simulink model "microgrid_phasor"  (R2025a)
settings: Solver=ode23tb  StartTime=0  StopTime=4253.748  RelTol=1e-4
libraries: spsGroundLib x3, spsThreePhaseParallelRLCBranchLib x1, spsThreePhaseDynamicLoadLib x1, spsThreePhaseSourceLib x1, spsThreePhaseVIMeasurementLib x1, spspowerguiLib x1
settings Model: Creator=daniellee  LastModifiedBy=daniellee

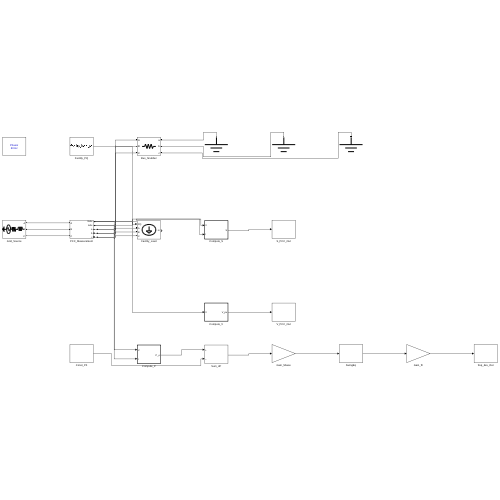
[thumbnail: Simulink's stored preview of the top-level diagram]
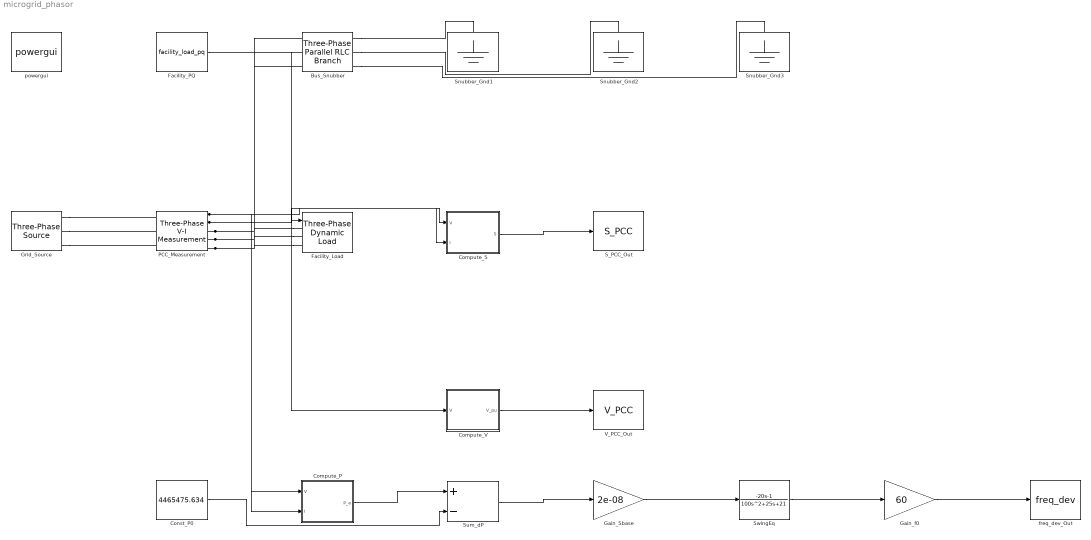
== system microgrid_phasor ==
  Bus_Snubber : spsThreePhaseParallelRLCBranchLib/Three-Phase Parallel RLC Branch  LConnTagsString=A|B|C  RConnTagsString=A|B|C  BranchType=R  Resistance=1e7  Inductance=1e9  Capacitance=1e-12  Measurements=None
  Compute_P : MATLAB Function  TreatAsAtomicUnit=on
  Compute_S : MATLAB Function  TreatAsAtomicUnit=on
  Compute_V : MATLAB Function  TreatAsAtomicUnit=on
  Const_P0 : Constant  Value=4465475.634
  Facility_Load : spsThreePhaseDynamicLoadLib/Three-Phase Dynamic Load  NominalVoltage=[25000 60]  ActiveReactivePowers=[4465475.634 1275123.081]  PositiveSequence=[0.994 -11.8]  ExternalControl=on  NpNq=[0 0]  TimeConstants="[0  0  0  0]"  MinimumVoltage=0.7  Tfilter=1e-4  LoadFlowParameters=[4,0,0,0,0]
      settings: LibrarySourceBlock=|
      | sps_lib/Passives/Three-Phase
      | Dynamic Load
  Facility_PQ : FromWorkspace  VariableName=facility_load_pq  OutputAfterFinalValue=Holding final value
  Gain_Sbase : Gain  Gain=2e-08
  Gain_f0 : Gain  Gain=60
  Grid_Source : spsThreePhaseSourceLib/Three-Phase Source  InternalConnection=Yg  VoltagePhases=off  Voltage=25000  PhaseAngle=0  Voltage_phases=[25e3 25e3 25e3]/sqrt(3)  PhaseAngles_phases=[0 -120 +120]  Frequency=60  NonIdealSource=on  SpecifyImpedance=on  Resistance=0.8929  Inductance=16.58e-3  ShortCircuitLevel=100000000  BaseVoltage=25000  XRratio=7  BusType=swing  Pref=10e3  Qref=0  Prefabc=[10e3, 10e3, 10e3]  Qrefabc=[0, 0, 0]  Qmin=-inf  Qmax=inf
  PCC_Measurement : spsThreePhaseVIMeasurementLib/Three-Phase V-I Measurement  VoltageMeasurement=phase-to-ground  SetLabelV=off  LabelV=Vabc  Vpu=off  VpuLL=off  CurrentMeasurement=yes  SetLabelI=off  LabelI=Iabc  Ipu=off  Pbase=100e6  Vbase=500e3  OutputType=Complex  PhasorSimulation=off  PSBequivalent=0
  S_PCC_Out : ToWorkspace  VariableName=S_PCC  SaveFormat=Timeseries  SampleTime=-1
  Snubber_Gnd1 : spsGroundLib/Ground  LConnTagsString=a
  Snubber_Gnd2 : spsGroundLib/Ground  LConnTagsString=a
  Snubber_Gnd3 : spsGroundLib/Ground  LConnTagsString=a
  Sum_dP : Sum  Inputs=+-
  SwingEq : TransferFcn  Numerator=[-20 -1]  Denominator=[100 25 21]
  V_PCC_Out : ToWorkspace  VariableName=V_PCC  SaveFormat=Timeseries  SampleTime=-1
  freq_dev_Out : ToWorkspace  VariableName=freq_dev  SaveFormat=Timeseries  SampleTime=-1
  powergui : spspowerguiLib/powergui  Priority=1  SimulationMode=Phasor  SampleTime=50e-6  frequency=60  Iterations=50  frequencyindice=60  Pbase=100e6  ErrMax=1e-4  UnitsV=kV  UnitsW=MW  buscounter=0  FunctionMessages=off  echomessages=off  EnableUseOfTLC=off  CurrentSourceSwitches=off  DisableSnubberDevices=off  DisableRonSwitches=off  DisableVfSwitches=off  DisplayEquations=off  AutomaticDiscreteSolvers=off  SolverType=Tustin/Backward Euler (TBE)  Interpol=off  ExternalGateDelay=off  methode=off  Ts=100  x0status=blocks  SPID=on  SwTol=0  HookPort=off  NonlinearTolerance=1e-4  nMaxIteration=100  ContinueOnMaxIteration=off  RestoreLinks=warning  ResistiveCurrentMeasurement=off  Frange=[0:2:500]  Ylog=off  Xlog=on  ShowGrid=off  save=off  variable=ZData  structure=0  ZoomFFT=off  StartTime=0.0  cycles=1  DisplayStyle=1  fundamental=60  FreqAxis=off  MaxFrequency=1000  frequencyindicesteady=1  RmsSteady=1  display=off
  wires:
  Facility_PQ/1 -> Facility_Load/1
  PCC_Measurement/1 -> Compute_S/1(V), Compute_V/1(V), Compute_P/1(V)
  PCC_Measurement/2 -> Compute_S/2(I), Compute_P/2(I)
  Compute_S/1(S) -> S_PCC_Out/1
  Compute_V/1(V_pu) -> V_PCC_Out/1
  Compute_P/1(P_e) -> Sum_dP/1
  Const_P0/1 -> Sum_dP/2
  Sum_dP/1 -> Gain_Sbase/1
  Gain_Sbase/1 -> SwingEq/1
  SwingEq/1 -> Gain_f0/1
  Gain_f0/1 -> freq_dev_Out/1
  connections:
  Grid_Source/RConn1 -- PCC_Measurement/LConn1
  Facility_Load/LConn1 -- PCC_Measurement/RConn1 -- Bus_Snubber/LConn1
  Grid_Source/RConn2 -- PCC_Measurement/LConn2
  Facility_Load/LConn2 -- PCC_Measurement/RConn2 -- Bus_Snubber/LConn2
  Grid_Source/RConn3 -- PCC_Measurement/LConn3
  Facility_Load/LConn3 -- PCC_Measurement/RConn3 -- Bus_Snubber/LConn3
  Bus_Snubber/RConn1 -- Snubber_Gnd1/LConn1
  Bus_Snubber/RConn2 -- Snubber_Gnd2/LConn1
  Bus_Snubber/RConn3 -- Snubber_Gnd3/LConn1

== matlab function microgrid_phasor/Compute_S ==
  data: V input; S output; I input
function S = compute_S(V, I)
%#codegen
% V, I: 3x1 complex PEAK phasors [a;b;c] in volts / amps.
% Three-phase complex power in VA (peak-phasor convention):
S = sum(V .* conj(I)) / 2;

== matlab function microgrid_phasor/Compute_P ==
  data: V input; P_e output; I input
function P_e = compute_P(V, I)
%#codegen
P_e = real(sum(V .* conj(I)) / 2);

== matlab function microgrid_phasor/Compute_V ==
  data: V input; V_pu output
function V_pu = compute_V(V)
%#codegen
% V: 3x1 complex PEAK phase-to-ground phasors from PCC measurement.
% Nominal peak phase voltage at 25000 V LL-rms: 20412.41452 V peak.
V_pu = mean(abs(V)) / 20412.41452;
